simulink model "Progetto_robotics_linear"  (R2021a)
settings: Solver=ode4  StartTime=0.0  StopTime=Tsim_lin  FixedStep=Ts  RelTol=1e-3
InitFcn:
  | I1=1;
  | I2=2;
  | I3 =3;
values from neighbouring files (symbols this model uses):
  q_iniz_lin = [-pi/4;+3/4*pi;-3/4*pi]    [File_main_lineare.m]
(part 2 of 2)

== matlab function Progetto_robotics_linear/q_quattrodot ==
  data: q input; qdot input; qdotdot input; q_triplodot input; alpha input; q_quattrodot output; y input; gain input
% THIS CODE COMPUTES THE FOURTH DERIVATIVE OF THE JOINT VARIABLES q BASED
% ON A CONSTRAINED OPTIMIZATION ALGORITHM

% UNCOMMENT EACH SECTION CORRESPONDING TO THE FOLLOWING SUBDIVISIONS

% CASE A1:   W=I   , tau_0=0
% CASE B1:   W=inv(M)   , tau_0=0
% CASE C1:   W=inv(M)^2   , tau_0=0

% CASE A2:   W=I   , tau_0!=0
% CASE B2:   W=inv(M)   , tau_0!=0
% CASE C2:   W=inv(M)^2   , tau_0!=0

%% CASE A1
% 
% function q_quattrodot = fcn(q,qdot,qdotdot,q_triplodot,alpha,y,gain)
% 
% q1=q(1);
% q2=q(2);
% q3=q(3);
% 
% q1_dot=qdot(1);
% q2_dot=qdot(2);
% q3_dot=qdot(3);
% 
% q1_dotdot=qdotdot(1);
% q2_dotdot=qdotdot(2);
% q3_dotdot=qdotdot(3);
% 
% q1_tridot=q_triplodot(1);
% q2_tridot=q_triplodot(2);
% q3_tridot=q_triplodot(3);
% 
% K=gain*[1,0,0;
%     0,1,0;
%     0,0,1];
% B=100*[1,0,0;
%     0,1,0;
%     0,0,1];
% 
% 
% M=[10*cos(q2 + q3) + 32*cos(q2) + 10*cos(q3) + 5049/100, 5*cos(q2 + q3) + 11*cos(q2) + 10*cos(q3) + 504/25, 5*cos(q2 + q3) + 5*cos(q3) + 583/100;
%    5*cos(q2 + q3) + 11*cos(q2) + 10*cos(q3) + 504/25,                              10*cos(q3) + 1133/50,                 10*cos(q3) + 583/100;
%                 5*cos(q2 + q3) + 5*cos(q3) + 583/100,                              10*cos(q3) + 583/100,                              583/100];
%               
%              
% 
%              
% J=[- sin(q1 + q2 + q3) - sin(q1 + q2) - sin(q1), - sin(q1 + q2 + q3) - sin(q1 + q2), -sin(q1 + q2 + q3);
%  cos(q1 + q2 + q3) + cos(q1 + q2) + cos(q1),   cos(q1 + q2 + q3) + cos(q1 + q2),  cos(q1 + q2 + q3)];
% 
% A=B*inv(K);
% W1=M*A^2*M;
% Jpinv=inv(W1)*transpose(J)*inv(J*inv(W1)*transpose(J)); 
% 
% q_quattrodot =-(eye(3)-Jpinv*J)*inv(M)*alpha + Jpinv *y;
% 


%% CASE B1
% 
% function q_quattrodot = fcn(q,qdot,qdotdot,q_triplodot,alpha,y,gain)
% 
% q1=q(1);
% q2=q(2);
% q3=q(3);
% 
% q1_dot=qdot(1);
% q2_dot=qdot(2);
% q3_dot=qdot(3);
% 
% q1_dotdot=qdotdot(1);
% q2_dotdot=qdotdot(2);
% q3_dotdot=qdotdot(3);
% 
% q1_tridot=q_triplodot(1);
% q2_tridot=q_triplodot(2);
% q3_tridot=q_triplodot(3);
% 
% K=gain*[1,0,0;
%     0,1,0;
%     0,0,1];
% B=100*[1,0,0;
%     0,1,0;
%     0,0,1];
% 
% 
% M=[10*cos(q2 + q3) + 32*cos(q2) + 10*cos(q3) + 5049/100, 5*cos(q2 + q3) + 11*cos(q2) + 10*cos(q3) + 504/25, 5*cos(q2 + q3) + 5*cos(q3) + 583/100;
%    5*cos(q2 + q3) + 11*cos(q2) + 10*cos(q3) + 504/25,                              10*cos(q3) + 1133/50,                 10*cos(q3) + 583/100;
%                 5*cos(q2 + q3) + 5*cos(q3) + 583/100,                              10*cos(q3) + 583/100,                              583/100];
%               
%              
% 
%              
% J=[- sin(q1 + q2 + q3) - sin(q1 + q2) - sin(q1), - sin(q1 + q2 + q3) - sin(q1 + q2), -sin(q1 + q2 + q3);
%  cos(q1 + q2 + q3) + cos(q1 + q2) + cos(q1),   cos(q1 + q2 + q3) + cos(q1 + q2),  cos(q1 + q2 + q3)];
% 
% % questa è la soluzione di donato
% % %q_quattrodot =-inv(M)*alpha+inv(M)*transpose(J)*inv(J*transpose(J))*J*alpha+transpose(J)*inv(J*transpose(J))*y;
% 
% %questa è la nostra soluzione
% J_pinv_minv=inv(M)*transpose(J)*inv(J*inv(M)*transpose(J));
% q_quattrodot =(J_pinv_minv*J-eye(3))*inv(M)*alpha+J_pinv_minv*y;
% 
% 



%% CASE C1
% function q_quattrodot = fcn(q,qdot,qdotdot,q_triplodot,alpha,y,gain)
% 
% q1=q(1);
% q2=q(2);
% q3=q(3);
% 
% q1_dot=qdot(1);
% q2_dot=qdot(2);
% q3_dot=qdot(3);
% 
% q1_dotdot=qdotdot(1);
% q2_dotdot=qdotdot(2);
% q3_dotdot=qdotdot(3);
% 
% q1_tridot=q_triplodot(1);
% q2_tridot=q_triplodot(2);
% q3_tridot=q_triplodot(3);
% 
% K=gain*[1,0,0;
%     0,1,0;
%     0,0,1];
% B=100*[1,0,0;
%     0,1,0;
%     0,0,1];
% 
% 
% M=[10*cos(q2 + q3) + 32*cos(q2) + 10*cos(q3) + 5049/100, 5*cos(q2 + q3) + 11*cos(q2) + 10*cos(q3) + 504/25, 5*cos(q2 + q3) + 5*cos(q3) + 583/100;
%    5*cos(q2 + q3) + 11*cos(q2) + 10*cos(q3) + 504/25,                              10*cos(q3) + 1133/50,                 10*cos(q3) + 583/100;
%                 5*cos(q2 + q3) + 5*cos(q3) + 583/100,                              10*cos(q3) + 583/100,                              583/100];
%               
%              
% 
%              
% J=[- sin(q1 + q2 + q3) - sin(q1 + q2) - sin(q1), - sin(q1 + q2 + q3) - sin(q1 + q2), -sin(q1 + q2 + q3);
%  cos(q1 + q2 + q3) + cos(q1 + q2) + cos(q1),   cos(q1 + q2 + q3) + cos(q1 + q2),  cos(q1 + q2 + q3)];
% 
% 
% q_quattrodot =-inv(M)*alpha+inv(M)*transpose(J)*inv(J*transpose(J))*J*alpha+transpose(J)*inv(J*transpose(J))*y;

% %% COPIA DEL VECCHIO CODICE DA BUTTARE 
% 
% 
%  
%           
%% CASE A2
function q_quattrodot = fcn(q,qdot,qdotdot,q_triplodot,alpha,y,gain)

q1=q(1);
q2=q(2);
q3=q(3);

q1_dot=qdot(1);
q2_dot=qdot(2);
q3_dot=qdot(3);

q1_dotdot=qdotdot(1);
q2_dotdot=qdotdot(2);
q3_dotdot=qdotdot(3);

q1_tridot=q_triplodot(1);
q2_tridot=q_triplodot(2);
q3_tridot=q_triplodot(3);

K=gain*[1,0,0;
    0,1,0;
    0,0,1];
B=100*[1,0,0;
    0,1,0;
    0,0,1];


M=[10*cos(q2 + q3) + 32*cos(q2) + 10*cos(q3) + 5049/100, 5*cos(q2 + q3) + 16*cos(q2) + 10*cos(q3) + 1133/50, 5*cos(q2 + q3) + 5*cos(q3) + 583/100;
  5*cos(q2 + q3) + 16*cos(q2) + 10*cos(q3) + 1133/50,                               10*cos(q3) + 1133/50,                  5*cos(q3) + 583/100;
               5*cos(q2 + q3) + 5*cos(q3) + 583/100,                                5*cos(q3) + 583/100,                              583/100];

J=[- sin(q1 + q2 + q3) - sin(q1 + q2) - sin(q1), - sin(q1 + q2 + q3) - sin(q1 + q2), -sin(q1 + q2 + q3);
 cos(q1 + q2 + q3) + cos(q1 + q2) + cos(q1),   cos(q1 + q2 + q3) + cos(q1 + q2),  cos(q1 + q2 + q3)];
              
             

% K_1=125*eye(3);             
% K_2=75*eye(3);      
% K_3=25*eye(3);  

% (s+5)^3
K_1=125*eye(3);             
K_2=75*eye(3);      
K_3=15*eye(3);  
tau_0=-K_1*[q1_dot;q2_dot;q3_dot]-K_2*[q1_dotdot;q2_dotdot;q3_dotdot]-K_3*[q1_tridot;q2_tridot;q3_tridot];       

A=B*inv(K);
             
Jpinv=inv(M*A^2*M)*transpose(J)*inv(J*inv(M*A^2*M)*transpose(J));

q_quattrodot =(eye(3)-Jpinv *J)*inv(M)*inv(A)*tau_0-(eye(3)-Jpinv *J)*inv(M)*alpha+Jpinv*y;       


% 
%% CASE B2

% function q_quattrodot = fcn(q,qdot,qdotdot,q_triplodot,alpha,y,gain)
% 
% q1=q(1);
% q2=q(2);
% q3=q(3);
% 
% q1_dot=qdot(1);
% q2_dot=qdot(2);
% q3_dot=qdot(3);
% 
% q1_dotdot=qdotdot(1);
% q2_dotdot=qdotdot(2);
% q3_dotdot=qdotdot(3);
% 
% q1_tridot=q_triplodot(1);
% q2_tridot=q_triplodot(2);
% q3_tridot=q_triplodot(3);
% 
% K=gain*[1,0,0;
%     0,1,0;
%     0,0,1];
% B=100*[1,0,0;
%     0,1,0;
%     0,0,1];
% 
% 
% M=[10*cos(q2 + q3) + 32*cos(q2) + 10*cos(q3) + 5049/100, 5*cos(q2 + q3) + 16*cos(q2) + 10*cos(q3) + 1133/50, 5*cos(q2 + q3) + 5*cos(q3) + 583/100;
%   5*cos(q2 + q3) + 16*cos(q2) + 10*cos(q3) + 1133/50,                               10*cos(q3) + 1133/50,                  5*cos(q3) + 583/100;
%                5*cos(q2 + q3) + 5*cos(q3) + 583/100,                                5*cos(q3) + 583/100,                              583/100];
% 
% J=[- sin(q1 + q2 + q3) - sin(q1 + q2) - sin(q1), - sin(q1 + q2 + q3) - sin(q1 + q2), -sin(q1 + q2 + q3);
%  cos(q1 + q2 + q3) + cos(q1 + q2) + cos(q1),   cos(q1 + q2 + q3) + cos(q1 + q2),  cos(q1 + q2 + q3)];
% 
% 
% % K_1=125*eye(3);             
% % K_2=75*eye(3);      
% % K_3=25*eye(3); 
% % 
% % % (s+10)^3
% % K_1=1000*eye(3);             
% % K_2=300*eye(3);      
% % K_3=30*eye(3);
% 
% % (s+10)^3
% K_1=8000*eye(3);             
% K_2=1200*eye(3);      
% K_3=60*eye(3);
% tau_0=-K_1*[q1_dot;q2_dot;q3_dot]-K_2*[q1_dotdot;q2_dotdot;q3_dotdot]-K_3*[q1_tridot;q2_tridot;q3_tridot];       
% 
% % soluzione di donato
% %q_quattrodot=-inv(M)*alpha+inv(M*B*inv(K))*tau_0+inv(M)*transpose(J)*inv(J*transpose(J))*J*alpha-inv(M*B*inv(K))*transpose(J)*inv(J*transpose(J))*J*tau_0+transpose(J)*inv(J*transpose(J))*y;
% 
% % soluzione nostra
% J_pinv_minv=inv(M)*transpose(J)*inv(J*inv(M)*transpose(J));
% q_quattrodot =(J_pinv_minv*J-eye(3))*inv(M)*alpha+J_pinv_minv*y+(eye(3)-J_pinv_minv*J)*inv(M)*inv(B*inv(K))*tau_0;
% % % 

% 
% 
%% CASE C2

% function q_quattrodot = fcn(q,qdot,qdotdot,q_triplodot,alpha,y,gain)
% 
% q1=q(1);
% q2=q(2);
% q3=q(3);
% 
% q1_dot=qdot(1);
% q2_dot=qdot(2);
% q3_dot=qdot(3);
% 
% q1_dotdot=qdotdot(1);
% q2_dotdot=qdotdot(2);
% q3_dotdot=qdotdot(3);
% 
% q1_tridot=q_triplodot(1);
% q2_tridot=q_triplodot(2);
% q3_tridot=q_triplodot(3);
% 
% K=gain*[1,0,0;
%     0,1,0;
%     0,0,1];
% B=100*[1,0,0;
%     0,1,0;
%     0,0,1];
% 
% 
% M=[10*cos(q2 + q3) + 32*cos(q2) + 10*cos(q3) + 5049/100, 5*cos(q2 + q3) + 16*cos(q2) + 10*cos(q3) + 1133/50, 5*cos(q2 + q3) + 5*cos(q3) + 583/100;
%   5*cos(q2 + q3) + 16*cos(q2) + 10*cos(q3) + 1133/50,                               10*cos(q3) + 1133/50,                  5*cos(q3) + 583/100;
%                5*cos(q2 + q3) + 5*cos(q3) + 583/100,                                5*cos(q3) + 583/100,                              583/100];
% 
% J=[- sin(q1 + q2 + q3) - sin(q1 + q2) - sin(q1), - sin(q1 + q2 + q3) - sin(q1 + q2), -sin(q1 + q2 + q3);
%  cos(q1 + q2 + q3) + cos(q1 + q2) + cos(q1),   cos(q1 + q2 + q3) + cos(q1 + q2),  cos(q1 + q2 + q3)];
%               
% 
% K_1=125*eye(3);             
% K_2=75*eye(3);      
% K_3=15*eye(3);    
% 
% 
% 
% tau_0=-K_1*[q1_dot;q2_dot;q3_dot]-K_2*[q1_dotdot;q2_dotdot;q3_dotdot]-K_3*[q1_tridot;q2_tridot;q3_tridot];       
% 
% q_quattrodot=-inv(M)*alpha+inv(B*inv(K)*M)*tau_0-transpose(J)*inv(J*transpose(J))*(-J*inv(M)*alpha+J*inv(B*inv(K)*M)*tau_0-y);

== matlab function Progetto_robotics_linear/alpha ==
  data: q input; alpha output; qdot input; qdotdot input; q_triplodot input; gain input
function alpha = fcn(q,qdot,qdotdot,q_triplodot,gain)

q1=q(1);
q2=q(2);
q3=q(3);

q1_dot=qdot(1);
q2_dot=qdot(2);
q3_dot=qdot(3);

q1_dotdot=qdotdot(1);
q2_dotdot=qdotdot(2);
q3_dotdot=qdotdot(3);

%usare per blocco jacobiano
q1_tridot=q_triplodot(1);
q2_tridot=q_triplodot(2);
q3_tridot=q_triplodot(3);


K=gain*eye(3);
B=100*[1,0,0;0,1,0;0,0,1];


%M matrix
m=[10*cos(q2 + q3) + 32*cos(q2) + 10*cos(q3) + 5049/100, 5*cos(q2 + q3) + 11*cos(q2) + 10*cos(q3) + 504/25, 5*cos(q2 + q3) + 5*cos(q3) + 583/100;
   5*cos(q2 + q3) + 11*cos(q2) + 10*cos(q3) + 504/25,                              10*cos(q3) + 1133/50,                 10*cos(q3) + 583/100;
                5*cos(q2 + q3) + 5*cos(q3) + 583/100,                              10*cos(q3) + 583/100,                              583/100];



%coriolis and centrif.
c=[- q1_dot*(q3_dot*(5*sin(q2 + q3) + 5*sin(q3)) + q2_dot*(5*sin(q2 + q3) + 16*sin(q2))) - q3_dot*(q1_dot*(5*sin(q2 + q3) + 5*sin(q3)) + q2_dot*(5*sin(q2 + q3) + 5*sin(q3)) + q3_dot*(5*sin(q2 + q3) + 5*sin(q3))) - q2_dot*(q3_dot*(5*sin(q2 + q3) + 5*sin(q3)) + q2_dot*(5*sin(q2 + q3) + 11*sin(q2)) + q1_dot*(5*sin(q2 + q3) + 16*sin(q2)));
                                                                                                                                                                                q1_dot*(q1_dot*(5*sin(q2 + q3) + 16*sin(q2)) - 5*q3_dot*sin(q3)) - q3_dot*(5*q1_dot*sin(q3) + 5*q2_dot*sin(q3) + 10*q3_dot*sin(q3)) - 5*q2_dot*q3_dot*sin(q3);
                                                                                                                                                                                                                               q1_dot*(q1_dot*(5*sin(q2 + q3) + 5*sin(q3)) + 5*q2_dot*sin(q3)) + q2_dot*(5*q1_dot*sin(q3) + 5*q2_dot*sin(q3))];



%coriolis and centrif. dotdot
cdotdot=[11*q2_dot^4*sin(q2) + 5*q3_dot^4*sin(q3) - 22*q2_dotdot^2*sin(q2) - 10*q3_dotdot^2*sin(q3) + 5*q2_dot^4*sin(q2 + q3) + 5*q3_dot^4*sin(q2 + q3) - 10*q2_dotdot^2*sin(q2 + q3) - 10*q3_dotdot^2*sin(q2 + q3) - 32*q1_dot*q2_tridot*sin(q2) - 32*q2_dot*q1_tridot*sin(q2) - 22*q2_dot*q2_tridot*sin(q2) - 10*q1_dot*q3_tridot*sin(q3) - 10*q3_dot*q1_tridot*sin(q3) - 10*q2_dot*q3_tridot*sin(q3) - 10*q3_dot*q2_tridot*sin(q3) - 10*q3_dot*q3_tridot*sin(q3) - 64*q1_dotdot*q2_dotdot*sin(q2) - 20*q1_dotdot*q3_dotdot*sin(q3) - 20*q2_dotdot*q3_dotdot*sin(q3) - 20*q2_dot^2*q1_dotdot*cos(q2 + q3) - 25*q2_dot^2*q2_dotdot*cos(q2 + q3) - 20*q3_dot^2*q1_dotdot*cos(q2 + q3) - 25*q2_dot^2*q3_dotdot*cos(q2 + q3) - 25*q3_dot^2*q2_dotdot*cos(q2 + q3) - 25*q3_dot^2*q3_dotdot*cos(q2 + q3) + 10*q1_dot*q2_dot^3*sin(q2 + q3) + 10*q1_dot*q3_dot^3*sin(q2 + q3) + 20*q2_dot*q3_dot^3*sin(q2 + q3) + 20*q2_dot^3*q3_dot*sin(q2 + q3) - 64*q2_dot^2*q1_dotdot*cos(q2) - 55*q2_dot^2*q2_dotdot*cos(q2) - 20*q3_dot^2*q1_dotdot*cos(q3) - 20*q3_dot^2*q2_dotdot*cos(q3) - 25*q3_dot^2*q3_dotdot*cos(q3) + 32*q1_dot*q2_dot^3*sin(q2) + 10*q1_dot*q3_dot^3*sin(q3) + 10*q2_dot*q3_dot^3*sin(q3) + 30*q2_dot^2*q3_dot^2*sin(q2 + q3) - 10*q1_dot*q2_tridot*sin(q2 + q3) - 10*q2_dot*q1_tridot*sin(q2 + q3) - 10*q1_dot*q3_tridot*sin(q2 + q3) - 10*q2_dot*q2_tridot*sin(q2 + q3) - 10*q3_dot*q1_tridot*sin(q2 + q3) - 10*q2_dot*q3_tridot*sin(q2 + q3) - 10*q3_dot*q2_tridot*sin(q2 + q3) - 10*q3_dot*q3_tridot*sin(q2 + q3) - 20*q1_dotdot*q2_dotdot*sin(q2 + q3) - 20*q1_dotdot*q3_dotdot*sin(q2 + q3) - 20*q2_dotdot*q3_dotdot*sin(q2 + q3) - 30*q1_dot*q2_dot*q2_dotdot*cos(q2 + q3) - 30*q1_dot*q2_dot*q3_dotdot*cos(q2 + q3) - 30*q1_dot*q3_dot*q2_dotdot*cos(q2 + q3) - 40*q2_dot*q3_dot*q1_dotdot*cos(q2 + q3) - 30*q1_dot*q3_dot*q3_dotdot*cos(q2 + q3) - 50*q2_dot*q3_dot*q2_dotdot*cos(q2 + q3) - 50*q2_dot*q3_dot*q3_dotdot*cos(q2 + q3) - 96*q1_dot*q2_dot*q2_dotdot*cos(q2) - 30*q1_dot*q3_dot*q3_dotdot*cos(q3) - 30*q2_dot*q3_dot*q3_dotdot*cos(q3) + 30*q1_dot*q2_dot*q3_dot^2*sin(q2 + q3) + 30*q1_dot*q2_dot^2*q3_dot*sin(q2 + q3);
                                                                                                                                                                                                                                                                                                                                                                                                                                                                                                                                                                                                                                                                                                                                                                                                                                                                                                                                                                                                                                                                                                                                10*q3_dot^4*sin(q3) + 32*q1_dotdot^2*sin(q2) - 20*q3_dotdot^2*sin(q3) + 10*q1_dotdot^2*sin(q2 + q3) + 32*q1_dot*q1_tridot*sin(q2) - 10*q1_dot*q3_tridot*sin(q3) - 10*q3_dot*q1_tridot*sin(q3) - 10*q2_dot*q3_tridot*sin(q3) - 10*q3_dot*q2_tridot*sin(q3) - 20*q3_dot*q3_tridot*sin(q3) - 20*q1_dotdot*q3_dotdot*sin(q3) - 20*q2_dotdot*q3_dotdot*sin(q3) + 5*q1_dot^2*q2_dotdot*cos(q2 + q3) + 5*q1_dot^2*q3_dotdot*cos(q2 + q3) + 16*q1_dot^2*q2_dotdot*cos(q2) - 20*q3_dot^2*q1_dotdot*cos(q3) - 20*q3_dot^2*q2_dotdot*cos(q3) - 50*q3_dot^2*q3_dotdot*cos(q3) + 10*q1_dot*q3_dot^3*sin(q3) + 10*q2_dot*q3_dot^3*sin(q3) - 5*q1_dot^2*q2_dot^2*sin(q2 + q3) - 5*q1_dot^2*q3_dot^2*sin(q2 + q3) - 16*q1_dot^2*q2_dot^2*sin(q2) + 10*q1_dot*q1_tridot*sin(q2 + q3) + 20*q1_dot*q2_dot*q1_dotdot*cos(q2 + q3) + 20*q1_dot*q3_dot*q1_dotdot*cos(q2 + q3) + 64*q1_dot*q2_dot*q1_dotdot*cos(q2) - 30*q1_dot*q3_dot*q3_dotdot*cos(q3) - 30*q2_dot*q3_dot*q3_dotdot*cos(q3) - 10*q1_dot^2*q2_dot*q3_dot*sin(q2 + q3);
                                                                                                                                                                                                                                                                                                                                                                                                                                                                                                                                                                                                                                                                                                                                                                                                                                                                                                                                                                                                                                                                                                                                                                                                                                                                                                                                                                                        10*q2_dotdot^2*sin(q3) + q1_tridot*(10*q1_dot*sin(q2 + q3) + 10*q1_dot*sin(q3) + 10*q2_dot*sin(q3)) + q3_dotdot*(5*q1_dot^2*cos(q3) + 5*q2_dot^2*cos(q3) + 5*q1_dot^2*cos(q2 + q3) + 10*q1_dot*q2_dot*cos(q3)) - q3_dot^2*(5*q1_dot^2*sin(q3) + 5*q2_dot^2*sin(q3) + 5*q1_dot^2*sin(q2 + q3) + 10*q1_dot*q2_dot*sin(q3)) + q1_dotdot^2*(10*sin(q2 + q3) + 10*sin(q3)) + 20*q1_dotdot*q2_dotdot*sin(q3) + 5*q1_dot^2*q2_dotdot*cos(q2 + q3) + 2*q3_dot*q1_dotdot*(10*q1_dot*cos(q2 + q3) + 10*q1_dot*cos(q3) + 10*q2_dot*cos(q3)) + q2_tridot*sin(q3)*(10*q1_dot + 10*q2_dot) - 5*q1_dot^2*q2_dot^2*sin(q2 + q3) + 2*q3_dot*q2_dotdot*cos(q3)*(10*q1_dot + 10*q2_dot) + 20*q1_dot*q2_dot*q1_dotdot*cos(q2 + q3) - 10*q1_dot^2*q2_dot*q3_dot*sin(q2 + q3)];
                                                                                                                                                                                                                                                                                                                                                                                                          
 




mdot=[- q3_dot*(10*sin(q2 + q3) + 10*sin(q3)) - q2_dot*(10*sin(q2 + q3) + 32*sin(q2)), - q2_dot*(5*sin(q2 + q3) + 11*sin(q2)) - q3_dot*(5*sin(q2 + q3) + 10*sin(q3)), - 5*q2_dot*sin(q2 + q3) - q3_dot*(5*sin(q2 + q3) + 5*sin(q3));
  - q2_dot*(5*sin(q2 + q3) + 11*sin(q2)) - q3_dot*(5*sin(q2 + q3) + 10*sin(q3)),                                                            -10*q3_dot*sin(q3),                                            -10*q3_dot*sin(q3);
                 - 5*q2_dot*sin(q2 + q3) - q3_dot*(5*sin(q2 + q3) + 5*sin(q3)),                                                            -10*q3_dot*sin(q3),                                                             0];
 

mdotdot=[(- 10*cos(q2 + q3) - 32*cos(q2))*q2_dot^2 - 20*cos(q2 + q3)*q2_dot*q3_dot + (- 10*cos(q2 + q3) - 10*cos(q3))*q3_dot^2 - q3_dotdot*(10*sin(q2 + q3) + 10*sin(q3)) - q2_dotdot*(10*sin(q2 + q3) + 32*sin(q2)), (- 5*cos(q2 + q3) - 11*cos(q2))*q2_dot^2 - 10*cos(q2 + q3)*q2_dot*q3_dot + (- 5*cos(q2 + q3) - 10*cos(q3))*q3_dot^2 - q2_dotdot*(5*sin(q2 + q3) + 11*sin(q2)) - q3_dotdot*(5*sin(q2 + q3) + 10*sin(q3)), - 5*cos(q2 + q3)*q2_dot^2 - 10*cos(q2 + q3)*q2_dot*q3_dot + (- 5*cos(q2 + q3) - 5*cos(q3))*q3_dot^2 - 5*q2_dotdot*sin(q2 + q3) - q3_dotdot*(5*sin(q2 + q3) + 5*sin(q3));
    (- 5*cos(q2 + q3) - 11*cos(q2))*q2_dot^2 - 10*cos(q2 + q3)*q2_dot*q3_dot + (- 5*cos(q2 + q3) - 10*cos(q3))*q3_dot^2 - q2_dotdot*(5*sin(q2 + q3) + 11*sin(q2)) - q3_dotdot*(5*sin(q2 + q3) + 10*sin(q3)),                                                                                                                                                            - 10*cos(q3)*q3_dot^2 - 10*q3_dotdot*sin(q3),                                                                                                                            - 10*cos(q3)*q3_dot^2 - 10*q3_dotdot*sin(q3);
                                    - 5*cos(q2 + q3)*q2_dot^2 - 10*cos(q2 + q3)*q2_dot*q3_dot + (- 5*cos(q2 + q3) - 5*cos(q3))*q3_dot^2 - 5*q2_dotdot*sin(q2 + q3) - q3_dotdot*(5*sin(q2 + q3) + 5*sin(q3)),                                                                                                                                                            - 10*cos(q3)*q3_dot^2 - 10*q3_dotdot*sin(q3),                                                                                                                                                                       0];
 
                                    
alpha = 2*mdot*[q1_tridot;q2_tridot;q3_tridot]+(mdotdot+K+K*inv(B)*m)*[q1_dotdot;q2_dotdot;q3_dotdot]+cdotdot+c ;

== matlab function Progetto_robotics_linear/q_triplodot ==
  data: q input; q_triplodot output; qdot input; qdotdot input; thetadot input; gain input
function q_triplodot = fcn(q,qdot,qdotdot,thetadot,gain)




q1=q(1);
q2=q(2);
q3=q(3);

q1_dot=qdot(1);
q2_dot=qdot(2);
q3_dot=qdot(3);

q1_dotdot=qdotdot(1);
q2_dotdot=qdotdot(2);
q3_dotdot=qdotdot(3);

tdot=[thetadot(1);thetadot(2);thetadot(3)];





%elastic matrix
K=gain*eye(3);


%M matrix
m=[10*cos(q2 + q3) + 32*cos(q2) + 10*cos(q3) + 5049/100, 5*cos(q2 + q3) + 11*cos(q2) + 10*cos(q3) + 504/25, 5*cos(q2 + q3) + 5*cos(q3) + 583/100;
   5*cos(q2 + q3) + 11*cos(q2) + 10*cos(q3) + 504/25,                              10*cos(q3) + 1133/50,                 10*cos(q3) + 583/100;
                5*cos(q2 + q3) + 5*cos(q3) + 583/100,                              10*cos(q3) + 583/100,                              583/100];


%coriolis and centrif. dot
cdot=[- 11*q2_dot^3*cos(q2) - 5*q3_dot^3*cos(q3) - 5*q2_dot^3*cos(q2 + q3) - 5*q3_dot^3*cos(q2 + q3) - 32*q1_dot*q2_dotdot*sin(q2) - 32*q2_dot*q1_dotdot*sin(q2) - 22*q2_dot*q2_dotdot*sin(q2) - 10*q1_dot*q3_dotdot*sin(q3) - 10*q3_dot*q1_dotdot*sin(q3) - 10*q2_dot*q3_dotdot*sin(q3) - 10*q3_dot*q2_dotdot*sin(q3) - 10*q3_dot*q3_dotdot*sin(q3) - 10*q1_dot*q2_dot^2*cos(q2 + q3) - 10*q1_dot*q3_dot^2*cos(q2 + q3) - 15*q2_dot*q3_dot^2*cos(q2 + q3) - 15*q2_dot^2*q3_dot*cos(q2 + q3) - 32*q1_dot*q2_dot^2*cos(q2) - 10*q1_dot*q3_dot^2*cos(q3) - 10*q2_dot*q3_dot^2*cos(q3) - 10*q1_dot*q2_dotdot*sin(q2 + q3) - 10*q2_dot*q1_dotdot*sin(q2 + q3) - 10*q1_dot*q3_dotdot*sin(q2 + q3) - 10*q2_dot*q2_dotdot*sin(q2 + q3) - 10*q3_dot*q1_dotdot*sin(q2 + q3) - 10*q2_dot*q3_dotdot*sin(q2 + q3) - 10*q3_dot*q2_dotdot*sin(q2 + q3) - 10*q3_dot*q3_dotdot*sin(q2 + q3) - 20*q1_dot*q2_dot*q3_dot*cos(q2 + q3);
                                                                                                                                                                                                                                                                                                                                                                                                                                                                                                         32*q1_dot*q1_dotdot*sin(q2) - 10*q3_dot^3*cos(q3) - 10*q1_dot*q3_dotdot*sin(q3) - 10*q3_dot*q1_dotdot*sin(q3) - 10*q2_dot*q3_dotdot*sin(q3) - 10*q3_dot*q2_dotdot*sin(q3) - 20*q3_dot*q3_dotdot*sin(q3) + 5*q1_dot^2*q2_dot*cos(q2 + q3) + 5*q1_dot^2*q3_dot*cos(q2 + q3) + 16*q1_dot^2*q2_dot*cos(q2) - 10*q1_dot*q3_dot^2*cos(q3) - 10*q2_dot*q3_dot^2*cos(q3) + 10*q1_dot*q1_dotdot*sin(q2 + q3);
                                                                                                                                                                                                                                                                                                                                                                                                                                                                                                                                                                                                                        q1_dotdot*(2*q1_dot*(5*sin(q2 + q3) + 5*sin(q3)) + 10*q2_dot*sin(q3)) + q2_dotdot*(10*q1_dot*sin(q3) + 10*q2_dot*sin(q3)) + q3_dot*(q1_dot*(q1_dot*(5*cos(q2 + q3) + 5*cos(q3)) + 5*q2_dot*cos(q3)) + q2_dot*(5*q1_dot*cos(q3) + 5*q2_dot*cos(q3))) + 5*q1_dot^2*q2_dot*cos(q2 + q3)];
 
  
                                                                                                                                                                                                    

mdot=[- q3_dot*(10*sin(q2 + q3) + 10*sin(q3)) - q2_dot*(10*sin(q2 + q3) + 32*sin(q2)), - q2_dot*(5*sin(q2 + q3) + 11*sin(q2)) - q3_dot*(5*sin(q2 + q3) + 10*sin(q3)), - 5*q2_dot*sin(q2 + q3) - q3_dot*(5*sin(q2 + q3) + 5*sin(q3));
  - q2_dot*(5*sin(q2 + q3) + 11*sin(q2)) - q3_dot*(5*sin(q2 + q3) + 10*sin(q3)),                                                            -10*q3_dot*sin(q3),                                            -10*q3_dot*sin(q3);
                 - 5*q2_dot*sin(q2 + q3) - q3_dot*(5*sin(q2 + q3) + 5*sin(q3)),                                                            -10*q3_dot*sin(q3),                                                             0];


q_triplodot = -inv(m)*(mdot*[q1_dotdot;q2_dotdot;q3_dotdot]+cdot+K*([q1_dot;q2_dot;q3_dot]-tdot));

== matlab function Progetto_robotics_linear/trajectory block ==
  data: t input; y output; q input; qdot input; qdotdot input; q_triplodot input
function y = fcn(t,q,qdot,qdotdot,q_triplodot)



q1=q(1);
q2=q(2);
q3=q(3);

q1_dot=qdot(1);
q2_dot=qdot(2);
q3_dot=qdot(3);

q1_dotdot=qdotdot(1);
q2_dotdot=qdotdot(2);
q3_dotdot=qdotdot(3);


q1_tridot=q_triplodot(1);
q2_tridot=q_triplodot(2);
q3_tridot=q_triplodot(3);


p=[cos(q1)+cos(q1+q2)+cos(q1+q2+q3);
    sin(q1)+sin(q1+q2)+sin(q1+q2+q3)];


%JACOBIANO
J=[- sin(q1 + q2 + q3) - sin(q1 + q2) - sin(q1), - sin(q1 + q2 + q3) - sin(q1 + q2), -sin(q1 + q2 + q3);
 cos(q1 + q2 + q3) + cos(q1 + q2) + cos(q1),   cos(q1 + q2 + q3) + cos(q1 + q2),  cos(q1 + q2 + q3)];


%JDOT
Jdot=[- q1_dot*(cos(q1 + q2 + q3) + cos(q1 + q2) + cos(q1)) - q3_dot*cos(q1 + q2 + q3) - q2_dot*(cos(q1 + q2 + q3) + cos(q1 + q2)), - q3_dot*cos(q1 + q2 + q3) - q1_dot*(cos(q1 + q2 + q3) + cos(q1 + q2)) - q2_dot*(cos(q1 + q2 + q3) + cos(q1 + q2)), -cos(q1 + q2 + q3)*(q1_dot + q2_dot + q3_dot);
- q2_dot*(sin(q1 + q2 + q3) + sin(q1 + q2)) - q1_dot*(sin(q1 + q2 + q3) + sin(q1 + q2) + sin(q1)) - q3_dot*sin(q1 + q2 + q3), - q1_dot*(sin(q1 + q2 + q3) + sin(q1 + q2)) - q2_dot*(sin(q1 + q2 + q3) + sin(q1 + q2)) - q3_dot*sin(q1 + q2 + q3), -sin(q1 + q2 + q3)*(q1_dot + q2_dot + q3_dot)];
 

%JDOTDOT
Jdotdot=[  q1_dot^2*(sin(q1 + q2 + q3) + sin(q1 + q2) + sin(q1)) + q3_dot^2*sin(q1 + q2 + q3) + q2_dot^2*(sin(q1 + q2 + q3) + sin(q1 + q2)) - q1_dotdot*(cos(q1 + q2 + q3) + cos(q1 + q2) + cos(q1)) - q3_dotdot*cos(q1 + q2 + q3) - q2_dotdot*(cos(q1 + q2 + q3) + cos(q1 + q2)) + 2*q1_dot*q3_dot*sin(q1 + q2 + q3) + 2*q2_dot*q3_dot*sin(q1 + q2 + q3) + 2*q1_dot*q2_dot*(sin(q1 + q2 + q3) + sin(q1 + q2)),   q3_dot^2*sin(q1 + q2 + q3) + q1_dot^2*(sin(q1 + q2 + q3) + sin(q1 + q2)) + q2_dot^2*(sin(q1 + q2 + q3) + sin(q1 + q2)) - q3_dotdot*cos(q1 + q2 + q3) - q1_dotdot*(cos(q1 + q2 + q3) + cos(q1 + q2)) - q2_dotdot*(cos(q1 + q2 + q3) + cos(q1 + q2)) + 2*q1_dot*q3_dot*sin(q1 + q2 + q3) + 2*q2_dot*q3_dot*sin(q1 + q2 + q3) + 2*q1_dot*q2_dot*(sin(q1 + q2 + q3) + sin(q1 + q2)),   sin(q1 + q2 + q3)*q1_dot^2 + 2*sin(q1 + q2 + q3)*q1_dot*q2_dot + 2*sin(q1 + q2 + q3)*q1_dot*q3_dot + sin(q1 + q2 + q3)*q2_dot^2 + 2*sin(q1 + q2 + q3)*q2_dot*q3_dot + sin(q1 + q2 + q3)*q3_dot^2 - q1_dotdot*cos(q1 + q2 + q3) - q2_dotdot*cos(q1 + q2 + q3) - q3_dotdot*cos(q1 + q2 + q3);
- q2_dotdot*(sin(q1 + q2 + q3) + sin(q1 + q2)) - q1_dot^2*(cos(q1 + q2 + q3) + cos(q1 + q2) + cos(q1)) - q3_dot^2*cos(q1 + q2 + q3) - q2_dot^2*(cos(q1 + q2 + q3) + cos(q1 + q2)) - q1_dotdot*(sin(q1 + q2 + q3) + sin(q1 + q2) + sin(q1)) - q3_dotdot*sin(q1 + q2 + q3) - 2*q1_dot*q3_dot*cos(q1 + q2 + q3) - 2*q2_dot*q3_dot*cos(q1 + q2 + q3) - 2*q1_dot*q2_dot*(cos(q1 + q2 + q3) + cos(q1 + q2)), - q1_dotdot*(sin(q1 + q2 + q3) + sin(q1 + q2)) - q2_dotdot*(sin(q1 + q2 + q3) + sin(q1 + q2)) - q3_dot^2*cos(q1 + q2 + q3) - q1_dot^2*(cos(q1 + q2 + q3) + cos(q1 + q2)) - q2_dot^2*(cos(q1 + q2 + q3) + cos(q1 + q2)) - q3_dotdot*sin(q1 + q2 + q3) - 2*q1_dot*q3_dot*cos(q1 + q2 + q3) - 2*q2_dot*q3_dot*cos(q1 + q2 + q3) - 2*q1_dot*q2_dot*(cos(q1 + q2 + q3) + cos(q1 + q2)), - cos(q1 + q2 + q3)*q1_dot^2 - 2*cos(q1 + q2 + q3)*q1_dot*q2_dot - 2*cos(q1 + q2 + q3)*q1_dot*q3_dot - cos(q1 + q2 + q3)*q2_dot^2 - 2*cos(q1 + q2 + q3)*q2_dot*q3_dot - cos(q1 + q2 + q3)*q3_dot^2 - q1_dotdot*sin(q1 + q2 + q3) - q2_dotdot*sin(q1 + q2 + q3) - q3_dotdot*sin(q1 + q2 + q3)];
 
%JTRIPLODOT
Jtriplodot=[q1_dot^3*cos(q1) + q1_dot^3*cos(q1 + q2 + q3) + q2_dot^3*cos(q1 + q2 + q3) + q3_dot^3*cos(q1 + q2 + q3) - q1_tridot*cos(q1 + q2) - q2_tridot*cos(q1 + q2) - q1_tridot*cos(q1) + q1_dot^3*cos(q1 + q2) + q2_dot^3*cos(q1 + q2) - q1_tridot*cos(q1 + q2 + q3) - q2_tridot*cos(q1 + q2 + q3) - q3_tridot*cos(q1 + q2 + q3) + 3*q1_dot*q1_dotdot*sin(q1) + 3*q1_dot*q2_dot^2*cos(q1 + q2) + 3*q1_dot^2*q2_dot*cos(q1 + q2) + 3*q1_dot*q1_dotdot*sin(q1 + q2 + q3) + 3*q1_dot*q2_dotdot*sin(q1 + q2 + q3) + 3*q2_dot*q1_dotdot*sin(q1 + q2 + q3) + 3*q1_dot*q3_dotdot*sin(q1 + q2 + q3) + 3*q2_dot*q2_dotdot*sin(q1 + q2 + q3) + 3*q3_dot*q1_dotdot*sin(q1 + q2 + q3) + 3*q2_dot*q3_dotdot*sin(q1 + q2 + q3) + 3*q3_dot*q2_dotdot*sin(q1 + q2 + q3) + 3*q3_dot*q3_dotdot*sin(q1 + q2 + q3) + 3*q1_dot*q2_dot^2*cos(q1 + q2 + q3) + 3*q1_dot^2*q2_dot*cos(q1 + q2 + q3) + 3*q1_dot*q3_dot^2*cos(q1 + q2 + q3) + 3*q1_dot^2*q3_dot*cos(q1 + q2 + q3) + 3*q2_dot*q3_dot^2*cos(q1 + q2 + q3) + 3*q2_dot^2*q3_dot*cos(q1 + q2 + q3) + 3*q1_dot*q1_dotdot*sin(q1 + q2) + 3*q1_dot*q2_dotdot*sin(q1 + q2) + 3*q2_dot*q1_dotdot*sin(q1 + q2) + 3*q2_dot*q2_dotdot*sin(q1 + q2) + 6*q1_dot*q2_dot*q3_dot*cos(q1 + q2 + q3), q1_dot^3*cos(q1 + q2 + q3) + q2_dot^3*cos(q1 + q2 + q3) + q3_dot^3*cos(q1 + q2 + q3) - q1_tridot*cos(q1 + q2) - q2_tridot*cos(q1 + q2) + q1_dot^3*cos(q1 + q2) + q2_dot^3*cos(q1 + q2) - q1_tridot*cos(q1 + q2 + q3) - q2_tridot*cos(q1 + q2 + q3) - q3_tridot*cos(q1 + q2 + q3) + 3*q1_dot*q2_dot^2*cos(q1 + q2) + 3*q1_dot^2*q2_dot*cos(q1 + q2) + 3*q1_dot*q1_dotdot*sin(q1 + q2 + q3) + 3*q1_dot*q2_dotdot*sin(q1 + q2 + q3) + 3*q2_dot*q1_dotdot*sin(q1 + q2 + q3) + 3*q1_dot*q3_dotdot*sin(q1 + q2 + q3) + 3*q2_dot*q2_dotdot*sin(q1 + q2 + q3) + 3*q3_dot*q1_dotdot*sin(q1 + q2 + q3) + 3*q2_dot*q3_dotdot*sin(q1 + q2 + q3) + 3*q3_dot*q2_dotdot*sin(q1 + q2 + q3) + 3*q3_dot*q3_dotdot*sin(q1 + q2 + q3) + 3*q1_dot*q2_dot^2*cos(q1 + q2 + q3) + 3*q1_dot^2*q2_dot*cos(q1 + q2 + q3) + 3*q1_dot*q3_dot^2*cos(q1 + q2 + q3) + 3*q1_dot^2*q3_dot*cos(q1 + q2 + q3) + 3*q2_dot*q3_dot^2*cos(q1 + q2 + q3) + 3*q2_dot^2*q3_dot*cos(q1 + q2 + q3) + 3*q1_dot*q1_dotdot*sin(q1 + q2) + 3*q1_dot*q2_dotdot*sin(q1 + q2) + 3*q2_dot*q1_dotdot*sin(q1 + q2) + 3*q2_dot*q2_dotdot*sin(q1 + q2) + 6*q1_dot*q2_dot*q3_dot*cos(q1 + q2 + q3), q1_dot^3*cos(q1 + q2 + q3) + q2_dot^3*cos(q1 + q2 + q3) + q3_dot^3*cos(q1 + q2 + q3) - q1_tridot*cos(q1 + q2 + q3) - q2_tridot*cos(q1 + q2 + q3) - q3_tridot*cos(q1 + q2 + q3) + 3*q1_dot*q1_dotdot*sin(q1 + q2 + q3) + 3*q1_dot*q2_dotdot*sin(q1 + q2 + q3) + 3*q2_dot*q1_dotdot*sin(q1 + q2 + q3) + 3*q1_dot*q3_dotdot*sin(q1 + q2 + q3) + 3*q2_dot*q2_dotdot*sin(q1 + q2 + q3) + 3*q3_dot*q1_dotdot*sin(q1 + q2 + q3) + 3*q2_dot*q3_dotdot*sin(q1 + q2 + q3) + 3*q3_dot*q2_dotdot*sin(q1 + q2 + q3) + 3*q3_dot*q3_dotdot*sin(q1 + q2 + q3) + 3*q1_dot*q2_dot^2*cos(q1 + q2 + q3) + 3*q1_dot^2*q2_dot*cos(q1 + q2 + q3) + 3*q1_dot*q3_dot^2*cos(q1 + q2 + q3) + 3*q1_dot^2*q3_dot*cos(q1 + q2 + q3) + 3*q2_dot*q3_dot^2*cos(q1 + q2 + q3) + 3*q2_dot^2*q3_dot*cos(q1 + q2 + q3) + 6*q1_dot*q2_dot*q3_dot*cos(q1 + q2 + q3);
q1_dot^3*sin(q1) + q1_dot^3*sin(q1 + q2 + q3) + q2_dot^3*sin(q1 + q2 + q3) + q3_dot^3*sin(q1 + q2 + q3) - q1_tridot*sin(q1 + q2) - q2_tridot*sin(q1 + q2) - q1_tridot*sin(q1) + q1_dot^3*sin(q1 + q2) + q2_dot^3*sin(q1 + q2) - q1_tridot*sin(q1 + q2 + q3) - q2_tridot*sin(q1 + q2 + q3) - q3_tridot*sin(q1 + q2 + q3) - 3*q1_dot*q1_dotdot*cos(q1) + 3*q1_dot*q2_dot^2*sin(q1 + q2) + 3*q1_dot^2*q2_dot*sin(q1 + q2) - 3*q1_dot*q1_dotdot*cos(q1 + q2 + q3) - 3*q1_dot*q2_dotdot*cos(q1 + q2 + q3) - 3*q2_dot*q1_dotdot*cos(q1 + q2 + q3) - 3*q1_dot*q3_dotdot*cos(q1 + q2 + q3) - 3*q2_dot*q2_dotdot*cos(q1 + q2 + q3) - 3*q3_dot*q1_dotdot*cos(q1 + q2 + q3) - 3*q2_dot*q3_dotdot*cos(q1 + q2 + q3) - 3*q3_dot*q2_dotdot*cos(q1 + q2 + q3) - 3*q3_dot*q3_dotdot*cos(q1 + q2 + q3) + 3*q1_dot*q2_dot^2*sin(q1 + q2 + q3) + 3*q1_dot^2*q2_dot*sin(q1 + q2 + q3) + 3*q1_dot*q3_dot^2*sin(q1 + q2 + q3) + 3*q1_dot^2*q3_dot*sin(q1 + q2 + q3) + 3*q2_dot*q3_dot^2*sin(q1 + q2 + q3) + 3*q2_dot^2*q3_dot*sin(q1 + q2 + q3) - 3*q1_dot*q1_dotdot*cos(q1 + q2) - 3*q1_dot*q2_dotdot*cos(q1 + q2) - 3*q2_dot*q1_dotdot*cos(q1 + q2) - 3*q2_dot*q2_dotdot*cos(q1 + q2) + 6*q1_dot*q2_dot*q3_dot*sin(q1 + q2 + q3), q1_dot^3*sin(q1 + q2 + q3) + q2_dot^3*sin(q1 + q2 + q3) + q3_dot^3*sin(q1 + q2 + q3) - q1_tridot*sin(q1 + q2) - q2_tridot*sin(q1 + q2) + q1_dot^3*sin(q1 + q2) + q2_dot^3*sin(q1 + q2) - q1_tridot*sin(q1 + q2 + q3) - q2_tridot*sin(q1 + q2 + q3) - q3_tridot*sin(q1 + q2 + q3) + 3*q1_dot*q2_dot^2*sin(q1 + q2) + 3*q1_dot^2*q2_dot*sin(q1 + q2) - 3*q1_dot*q1_dotdot*cos(q1 + q2 + q3) - 3*q1_dot*q2_dotdot*cos(q1 + q2 + q3) - 3*q2_dot*q1_dotdot*cos(q1 + q2 + q3) - 3*q1_dot*q3_dotdot*cos(q1 + q2 + q3) - 3*q2_dot*q2_dotdot*cos(q1 + q2 + q3) - 3*q3_dot*q1_dotdot*cos(q1 + q2 + q3) - 3*q2_dot*q3_dotdot*cos(q1 + q2 + q3) - 3*q3_dot*q2_dotdot*cos(q1 + q2 + q3) - 3*q3_dot*q3_dotdot*cos(q1 + q2 + q3) + 3*q1_dot*q2_dot^2*sin(q1 + q2 + q3) + 3*q1_dot^2*q2_dot*sin(q1 + q2 + q3) + 3*q1_dot*q3_dot^2*sin(q1 + q2 + q3) + 3*q1_dot^2*q3_dot*sin(q1 + q2 + q3) + 3*q2_dot*q3_dot^2*sin(q1 + q2 + q3) + 3*q2_dot^2*q3_dot*sin(q1 + q2 + q3) - 3*q1_dot*q1_dotdot*cos(q1 + q2) - 3*q1_dot*q2_dotdot*cos(q1 + q2) - 3*q2_dot*q1_dotdot*cos(q1 + q2) - 3*q2_dot*q2_dotdot*cos(q1 + q2) + 6*q1_dot*q2_dot*q3_dot*sin(q1 + q2 + q3), q1_dot^3*sin(q1 + q2 + q3) + q2_dot^3*sin(q1 + q2 + q3) + q3_dot^3*sin(q1 + q2 + q3) - q1_tridot*sin(q1 + q2 + q3) - q2_tridot*sin(q1 + q2 + q3) - q3_tridot*sin(q1 + q2 + q3) - 3*q1_dot*q1_dotdot*cos(q1 + q2 + q3) - 3*q1_dot*q2_dotdot*cos(q1 + q2 + q3) - 3*q2_dot*q1_dotdot*cos(q1 + q2 + q3) - 3*q1_dot*q3_dotdot*cos(q1 + q2 + q3) - 3*q2_dot*q2_dotdot*cos(q1 + q2 + q3) - 3*q3_dot*q1_dotdot*cos(q1 + q2 + q3) - 3*q2_dot*q3_dotdot*cos(q1 + q2 + q3) - 3*q3_dot*q2_dotdot*cos(q1 + q2 + q3) - 3*q3_dot*q3_dotdot*cos(q1 + q2 + q3) + 3*q1_dot*q2_dot^2*sin(q1 + q2 + q3) + 3*q1_dot^2*q2_dot*sin(q1 + q2 + q3) + 3*q1_dot*q3_dot^2*sin(q1 + q2 + q3) + 3*q1_dot^2*q3_dot*sin(q1 + q2 + q3) + 3*q2_dot*q3_dot^2*sin(q1 + q2 + q3) + 3*q2_dot^2*q3_dot*sin(q1 + q2 + q3) + 6*q1_dot*q2_dot*q3_dot*sin(q1 + q2 + q3)];





p_in=[1.41;-0.41];
p_fin=[1.41;0.41];

h=norm(p_fin-p_in);
T=2.58;

s=h*(-20*(t/T)^7+70*(t/T)^6-84*(t/T)^5+35*(t/T)^4);

s_1=140*h/T*(-(t/T)^6+3*(t/T)^5-3*(t/T)^4+(t/T)^3);

s_2=420*h/T^2*(-2*(t/T)^5+5*(t/T)^4-4*(t/T)^3+(t/T)^2);

s_3=840*h/T^3*(-5*(t/T)^4+10*(t/T)^3-6*(t/T)^2+(t/T));

s_4=840*h/T^4*(-20*(t/T)^3+30*(t/T)^2-12*(t/T)+1);


r=p_in+s/h*(p_fin-p_in);

r_1=s_1/h*(p_fin-p_in);

r_2=s_2/h*(p_fin-p_in);
 
r_3=s_3/h*(p_fin-p_in);

r_4=s_4/h*(p_fin-p_in);

p_3=J*q_triplodot+2*Jdot*qdotdot+Jdotdot*qdot;
p_2=Jdot*qdot+J*qdotdot;
p_1=J*qdot;

% caso con (s+10)^2*(s+5)^2
K_0=2500*eye(2);
K_1=1500*eye(2);
K_2=325*eye(2);
K_3=30*eye(2);



X=r_4+K_3*(r_3-p_3)+K_2*(r_2-p_2)+K_1*(r_1-p_1)+K_0*(r-p);

y = X-3*Jdot*[q1_tridot;q2_tridot;q3_tridot]-2*Jdotdot*[q1_dotdot;q2_dotdot;q3_dotdot]-Jtriplodot*[q1_dot;q2_dot;q3_dot];

== matlab function Progetto_robotics_linear/  M_inversa1 ==
  data: q input; qdotdot output; ingresso input
function qdotdot = M_inversa(q,ingresso)


q1=q(1);
q2=q(2);
q3=q(3);
M=[10*cos(q2 + q3) + 32*cos(q2) + 10*cos(q3) + 5049/100, 5*cos(q2 + q3) + 11*cos(q2) + 10*cos(q3) + 504/25, 5*cos(q2 + q3) + 5*cos(q3) + 583/100;
   5*cos(q2 + q3) + 11*cos(q2) + 10*cos(q3) + 504/25,                              10*cos(q3) + 1133/50,                 10*cos(q3) + 583/100;
                5*cos(q2 + q3) + 5*cos(q3) + 583/100,                              10*cos(q3) + 583/100,                              583/100];




qdotdot = inv(M)*ingresso;
